simulink model "torque"  (R2018b)
settings: Solver=VariableStepAuto  StartTime=0.0  StopTime=10  RelTol=1e-3
values from neighbouring files (symbols this model uses):
  A = [0,1,0,0;-ks/Il,-cl/Il,ks/Il,0;0,0,0,1;ks/Im,0,-ks/Im,-cm/Im]    [base_mix.m]    (also in optimal_control.m)
  B = [0,0;0,1/Il;0,0;K/Im,0]    [base_mix.m]    (also in optimal_control.m)
  C = [0,0,1,0;1,0,0,0;-ks,0,ks,0]    [base_mix.m]    (also in optimal_control.m)
  D = zeros(3,2)    [base_mix.m]    (also in optimal_control.m)
  Kd = (2*ksai_torque*wn_torque+beta_torque)/den    [base_mix.m]
  Ki = (beta_torque*wn_torque^2)/den    [base_mix.m]
  Kp = ((2*ksai_torque*wn_torque*beta_torque+wn_torque^2-(Il+Im)*ks/Il/Im))/den    [base_mix.m]
libraries: simulink x1, cstblocks x1
settings Model: Creator=78224  LastModifiedBy=78224

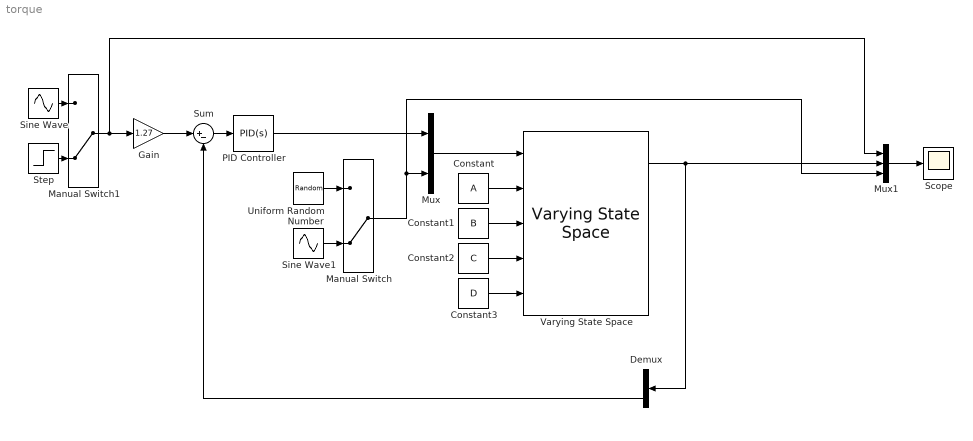
== system torque ==
  Constant : Constant  Value=A  VectorParams1D=off
  Constant1 : Constant  Value=B  VectorParams1D=off
  Constant2 : Constant  Value=C  VectorParams1D=off
  Constant3 : Constant  Value=D  VectorParams1D=off
  Demux : Demux  Outputs=3
  Gain : Gain  Gain=1.27
  Manual Switch : ManualSwitch  CurrentSetting=0
  Manual Switch1 : ManualSwitch  CurrentSetting=0
  Mux : Mux  Inputs=2
  Mux1 : Mux  Inputs=3
  PID Controller : simulink/Continuous/PID Controller  Controller=PID  Form=Parallel  TimeDomain=Continuous-time  SampleTime=-1  IntegratorMethod=Forward Euler  FilterMethod=Forward Euler  ControllerParametersSource=internal  P=Kp  I=Ki  D=Kd  UseFilter=on  N=100  TunerSelectOption=Transfer Function Based (PID Tuner App)  InitialConditionSource=internal  InitialConditionForIntegrator=0  InitialConditionForFilter=0  DifferentiatorICPrevScaledInput=0  ExternalReset=none  TrackingMode=off  Kt=1  LimitOutput=off  UpperSaturationLimit=inf  LowerSaturationLimit=-inf  LinearizeAsGain=on  AntiWindupMode=none  Kb=1  POutMin=[]  POutMax=[]  IOutMin=[]  IOutMax=[]  DOutMin=[]  DOutMax=[]  NOutMin=[]  NOutMax=[]  SumOutMin=[]  SumOutMax=[]  SaturationOutMin=[]  SaturationOutMax=[]  PParamMin=[]  PParamMax=[]  IParamMin=[]  IParamMax=[]  DParamMin=[]  DParamMax=[]  NParamMin=[]  NParamMax=[]  KbParamMin=[]  KbParamMax=[]  KtParamMin=[]  KtParamMax=[]  KbOutMin=[]  KbOutMax=[]  KtOutMin=[]  KtOutMax=[]  IntegratorOutMin=[]  IntegratorOutMax=[]  FilterOutMin=[]  FilterOutMax=[]  SumI1OutMin=[]  SumI1OutMax=[]  SumI2OutMin=[]  SumI2OutMax=[]  SumI3OutMin=[]  SumI3OutMax=[]  SumI4OutMin=[]  SumI4OutMax=[]  SumDOutMin=[]  SumDOutMax=[]  DifferentiatorOutMin=[]  DifferentiatorOutMax=[]  FilterDiffOutCoefMin=[]  FilterDiffOutCoefMax=[]  ReciprocalOutMin=[]  ReciprocalOutMax=[]  SumDenOutMin=[]  SumDenOutMax=[]  SumNumOutMin=[]  SumNumOutMax=[]  DivideOutMin=[]  DivideOutMax=[]  IntegratorContinuousStateAttributes=''  IntegratorStateMustResolveToSignalObject=off  IntegratorRTWStateStorageClass=Auto  FilterContinuousStateAttributes=''  FilterStateMustResolveToSignalObject=off  FilterRTWStateStorageClass=Auto  ParallelPVariant=InternalParameters  IdealPVariant=Disabled  IVariant=InternalParameters  DVariant=InternalParameters  IntegratorVariant=Continuous  SatVariant=Disabled  AWVariant=Passthrough  PCopyVariant=Disabled  TRVariant=Disabled  FdbkBlocksVariant=Forward  IdealPFdbkVariant=Disabled  SatFdbkVariant=Disabled  DerivativeFilterVariant=ContFilter  NVariant=InternalParameters  NCopyVariant=Disabled  FilterICVariant=InternalICsFilter  IntegratorICVariant=InternalICs  ExternalResetVariant=Disabled  TRSumVariant=Passthrough  SumFdbkVariant=Disabled  SumVariant=Sum_PID
  Scope : Scope
  Sine Wave : Sin  Amplitude=0  Frequency=2*pi*0.2  SampleTime=0
  Sine Wave1 : Sin  Amplitude=0  Frequency=2*pi*0.2  SampleTime=0
  Step : Step  SampleTime=0
  Sum : Sum  Inputs=|+-
  Uniform Random Number : UniformRandomNumber  SampleTime=0.1
  Varying State Space : cstblocks/Linear Parameter Varying/Varying State Space  x0=0  xNames=''  OutputX=on  OutputDX=on
      settings: SourceProductName=Control System Toolbox
  wires:
  Constant/1 -> Varying State Space/2
  Constant1/1 -> Varying State Space/3
  Constant2/1 -> Varying State Space/4
  Constant3/1 -> Varying State Space/5
  Mux1/1 -> Scope/1
  Mux/1 -> Varying State Space/1
  Manual Switch/1 -> Mux1/3, Mux/2
  Manual Switch1/1 -> Gain/1, Mux1/1
  Sum/1 -> PID Controller/1
  Varying State Space/1 -> Demux/1, Mux1/2
  Uniform Random Number/1 -> Manual Switch/1
  Sine Wave1/1 -> Manual Switch/2
  Step/1 -> Manual Switch1/2
  Sine Wave/1 -> Manual Switch1/1
  PID Controller/1 -> Mux/1
  Demux/3 -> Sum/2
  Gain/1 -> Sum/1
